simulink model "model2_controlable"  (R2024a)
settings: Solver=VariableStepAuto  StartTime=0.0  StopTime=10.0  RelTol=1e-3
settings Model: Creator=Professional  LastModifiedBy=Professional

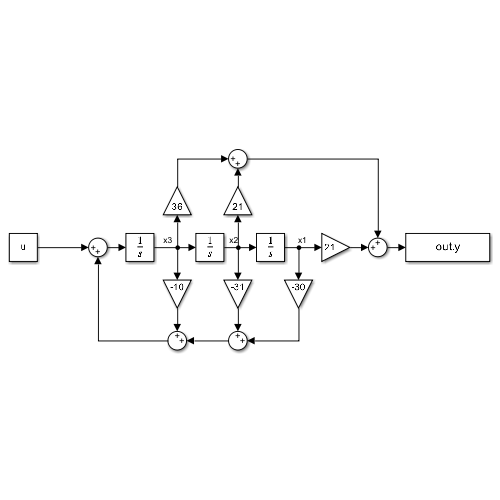
[thumbnail: Simulink's stored preview of the top-level diagram]
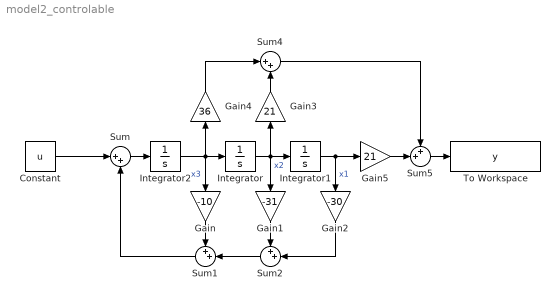
== system model2_controlable ==
  Constant : Constant  Value=u  SampleTime=0.0001
  Gain : Gain  Gain=-10
  Gain1 : Gain  Gain=-31
  Gain2 : Gain  Gain=-30
  Gain3 : Gain  Gain=21
  Gain4 : Gain  Gain=36
  Gain5 : Gain  Gain=21
  Integrator : Integrator
  Integrator1 : Integrator
  Integrator2 : Integrator
  Sum : Sum  Inputs=|++
  Sum1 : Sum  Inputs=++|
  Sum2 : Sum  Inputs=++|
  Sum4 : Sum  Inputs=|++
  Sum5 : Sum  Inputs=++|
  To Workspace : ToWorkspace  VariableName=y  SaveFormat=Timeseries  SampleTime=-1
  wires:
  Constant/1 -> Sum/1
  Sum/1 -> Integrator2/1
  Integrator/1 -> Gain3/1, Integrator1/1, Gain1/1  "x2"
  Gain/1 -> Sum1/1
  Gain1/1 -> Sum2/1
  Sum2/1 -> Sum1/2
  Sum1/1 -> Sum/2
  Gain2/1 -> Sum2/2
  Integrator1/1 -> Gain5/1, Gain2/1  "x1"
  Gain3/1 -> Sum4/2
  Gain4/1 -> Sum4/1
  Gain5/1 -> Sum5/2
  Sum5/1 -> To Workspace/1
  Sum4/1 -> Sum5/1
  Integrator2/1 -> Gain/1, Integrator/1, Gain4/1  "x3"
